simulink model "SingleStreamSSR"  (R2023a)
settings: Solver=VariableStepAuto  StartTime=0.0  StopTime=4096  RelTol=1e-3
PreLoadFcn:
  | xmcCheckSlxPath(bdroot)
  | SSR4_init
InitFcn:
  | xmcCheckSlxPath(bdroot)
  | SSR4_init;
undefined symbols (not defined in the file): FIR_MultiKernel_cin, FIR_MultiKernel_cincout, FIR_MultiKernel_cout, N, S, SHIFT_ACC, SingleStream, Taps, vsva2197, xcvc1902
libraries: aieBasic x40, aieUtilities x8, dspsrcs4 x1, simulink x1, vmcUtilities x1
(part 3 of 3)

== matlab function SingleStreamSSR/ComplexSource4/MATLAB Function ==
  data: u input; y1 output; y2 output; y3 output; y4 output
function [y1,y2,y3,y4] = fcn(u)

y1 = u(1:4:end);
y2 = u(2:4:end);
y3 = u(3:4:end);
y4 = u(4:4:end);
